simulink model "iqcomplete2_fixed"  (R2015a)
settings: Solver=FixedStepDiscrete  SolverMode=SingleTasking  StartTime=0.0  StopTime=1e-6  RelTol=1e-3
InitFcn:
  | Iamplitude = 0.8;
  | omega = 100e6;
  | betai = 2;
  | betaq = 3;
  | offsetdegree = -30;
  | Qradian = (90+offsetdegree)*pi/180;
  | WSize = 10;
undefined symbols (not defined in the file or in its folder): Newton, Raphson
libraries: dspsrcs4 x2
CloseFcn:
  | clear all
  | clc
settings Model: Creator=DPu1  LastModifiedBy=Karol
settings DataIOCC: SignalLoggingSaveFormat=ModelDataLogs  SaveOutput=off  SignalLogging=off  SaveTime=off
settings OptimizationCC: BlockReduction=off  ConditionallyExecuteInputs=off  InlineParams=on
settings DebuggingCC: AlgebraicLoopMsg=error  UnderspecifiedInitializationDetection=Classic  MergeDetectMultiDrivingBlocksExec=none  SolverPrmCheckMsg=warning  MultiTaskDSMMsg=warning  MultiTaskCondExecSysMsg=none  SingleTaskRateTransMsg=error  ParameterPrecisionLossMsg=none  StateNameClashWarn=warning
settings HardwareCC: ProdHWDeviceType=ASIC/FPGA->ASIC/FPGA  ProdEqTarget=off

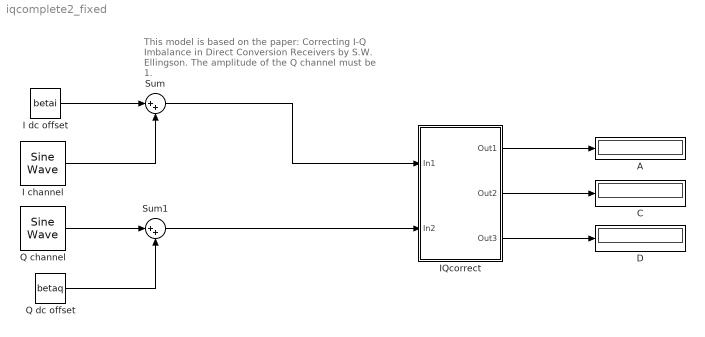
== system iqcomplete2_fixed ==
  note: This model is based on the paper:
      | Correcting I-Q Imbalance in Direct Conversion
      | Receivers by S.W. Ellingson.
      | The amplitude of the Q channel must be 1.
  A : Display
  C : Display
  D : Display
  I channel : dspsrcs4/Sine Wave  Amplitude=Iamplitude  Frequency=omega  Phase=0  SampleMode=Discrete  OutComplex=Real  CompMethod=Table lookup  TableSize=Speed  SampleTime=1/(1000e6)  SamplesPerFrame=1  ResetState=Restart at time zero  dataType=Fixed-point  wordLen=16  udDataType=sfix(16)  fracBitsMode=User-defined  numFracBits=15  OutDataTypeStr=fixdt(1,16,15)  LastOutDataTypeStr=fixdt(1,16,15)
  I dc offset : Constant  Value=betai  OutDataTypeStr=fixdt(1,16,0)  SampleTime=1/(1000e6)
  IQcorrect : Subsystem
  Q channel : dspsrcs4/Sine Wave  Amplitude=1  Frequency=omega  Phase=Qradian  SampleMode=Discrete  OutComplex=Real  CompMethod=Table lookup  TableSize=Speed  SampleTime=1/(1000e6)  SamplesPerFrame=1  ResetState=Restart at time zero  dataType=Fixed-point  wordLen=16  udDataType=sfix(16)  fracBitsMode=User-defined  numFracBits=14  OutDataTypeStr=fixdt(1,16,14)  LastOutDataTypeStr=fixdt(1,16,14)
  Q dc offset : Constant  Value=betaq  OutDataTypeStr=fixdt(1,16,0)  SampleTime=1/(1000e6)
  Sum : Sum  Inputs=|++  OutDataTypeStr=fixdt(1,16,13)
  Sum1 : Sum  Inputs=|++  OutDataTypeStr=fixdt(1,16,13)
  wires:
  Q channel/1 -> Sum1/1
  Q dc offset/1 -> Sum1/2
  IQcorrect/1(Out1) -> A/1
  IQcorrect/2(Out2) -> C/1
  IQcorrect/3(Out3) -> D/1
  I dc offset/1 -> Sum/1
  I channel/1 -> Sum/2
  Sum/1 -> IQcorrect/1(In1)
  Sum1/1 -> IQcorrect/2(In2)

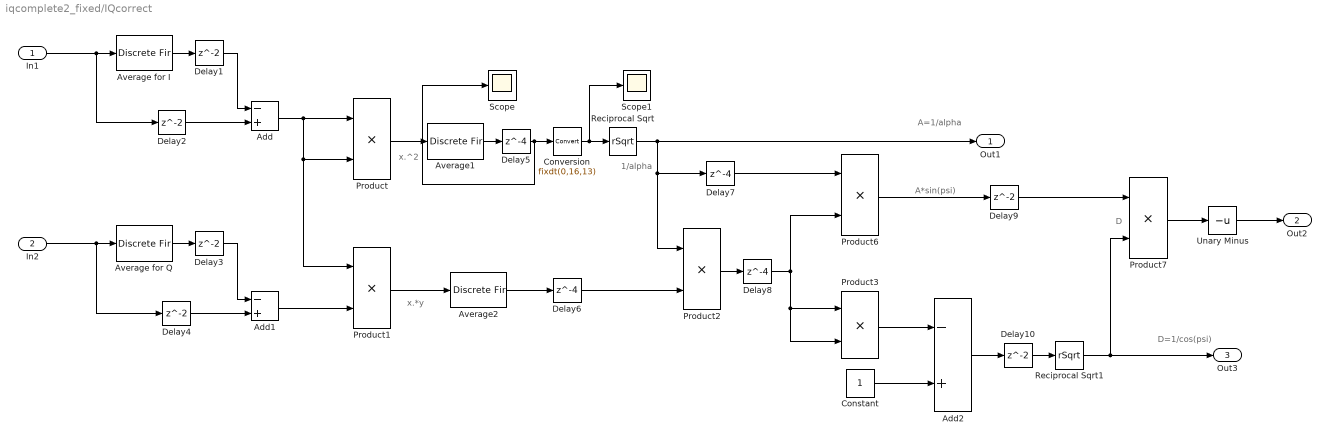
== system iqcomplete2_fixed/IQcorrect ==
  note: A*sin(psi)
  note: D
  note: D=1/cos(psi)
  note: A=1/alpha
  note: 1/alpha
  note: x.*y
  note: x.^2
  In1 : Inport
  In2 : Inport  Port=2
  Add : Sum  Inputs=-+  OutDataTypeStr=fixdt(1,16,15)
  Add1 : Sum  Inputs=-+  OutDataTypeStr=fixdt(1,16,15)
  Add2 : Sum  Inputs=-+  OutDataTypeStr=fixdt(0,16,15)
  Average for I : DiscreteFir  FilterStructure=Direct form transposed  Coefficients=ones(1,WSize)./WSize  OutDataTypeStr=fixdt(1,16,10)
  Average for Q : DiscreteFir  FilterStructure=Direct form transposed  Coefficients=ones(1,WSize)./WSize  OutDataTypeStr=fixdt(1,16,9)
  Average1 : DiscreteFir  FilterStructure=Direct form transposed  Coefficients=ones(1,WSize).*(2/WSize)  OutDataTypeStr=fixdt(1,16,12)
  Average2 : DiscreteFir  FilterStructure=Direct form transposed  Coefficients=ones(1,WSize).*(2/WSize)  OutDataTypeStr=fixdt(1,16,13)
  Constant : Constant  OutDataTypeStr=fixdt(1,16,0)  SampleTime=1/(1000e6)
  Conversion : DataTypeConversion  OutDataTypeStr=fixdt(0,16,13)
  Delay{1..4,9..10} (6 alike) : Delay  InitialCondition=0
  Delay{5..8} (4 alike) : Delay  DelayLength=4  InitialCondition=0
  Product : Product  OutDataTypeStr=fixdt(1,16,15)  RndMeth=Zero
  Product1 : Product  OutDataTypeStr=fixdt(1,16,15)  RndMeth=Zero
  Product2 : Product  OutDataTypeStr=fixdt(1,16,15)  RndMeth=Zero
  Product3 : Product  OutDataTypeStr=fixdt(0,16,16)  RndMeth=Zero
  Product6 : Product  OutDataTypeStr=fixdt(1,16,14)  RndMeth=Zero
  Product7 : Product  OutDataTypeStr=fixdt(1,16,14)  RndMeth=Zero
  Reciprocal Sqrt : Sqrt  Operator=rSqrt  OutDataTypeStr=fixdt(1,16,14)  IntermediateResultsDataTypeStr=Inherit: Inherit from input  AlgorithmType=Newton-Raphson  SaturateOnIntegerOverflow=on
  Reciprocal Sqrt1 : Sqrt  Operator=rSqrt  OutDataTypeStr=fixdt(0,16,15)  IntermediateResultsDataTypeStr=Inherit: Inherit from input  AlgorithmType=Newton-Raphson  SaturateOnIntegerOverflow=on
  Scope : Scope
  Scope1 : Scope
  Unary Minus : UnaryMinus
  Out1 : Outport
  Out2 : Outport  Port=2
  Out3 : Outport  Port=3
  wires:
  In2/1 -> Delay4/1, Average for Q/1
  Product3/1 -> Add2/1
  In1/1 -> Delay2/1, Average for I/1
  Product/1 -> Average1/1
  Add1/1 -> Product1/2
  Product2/1 -> Delay8/1
  Constant/1 -> Add2/2
  Add/1 -> Product1/1, Product/2, Product/1
  Product6/1 -> Delay9/1
  Product1/1 -> Average2/1
  Average1/1 -> Delay5/1
  Add2/1 -> Delay10/1
  Reciprocal Sqrt/1 -> Out1/1, Product2/1, Delay7/1
  Average2/1 -> Delay6/1
  Product7/1 -> Unary Minus/1
  Delay1/1 -> Add/1
  Delay2/1 -> Add/2
  Delay3/1 -> Add1/1
  Delay4/1 -> Add1/2
  Delay6/1 -> Product2/2
  Delay9/1 -> Product7/1
  Delay10/1 -> Reciprocal Sqrt1/1
  Delay7/1 -> Product6/1
  Delay8/1 -> Product6/2, Product3/2, Product3/1
  Unary Minus/1 -> Out2/1
  Average for I/1 -> Delay1/1
  Average for Q/1 -> Delay3/1
  Reciprocal Sqrt1/1 -> Product7/2, Out3/1
  Conversion/1 -> Scope1/1, Reciprocal Sqrt/1
  Delay5/1 -> Scope/1, Conversion/1
